simulink model "Closed_Loop_Simulation"  (R2022b)
settings: Solver=VariableStepAuto  StartTime=0.0  StopTime=100  RelTol=1e-3
values from neighbouring files (symbols this model uses):
  den = conv([2 1 0],[10 1])    [LAB03.m]    (also in StaticVelocityErrorConstant.m = [1 0])
  num = [2.5 5]    [LAB03.m]    (also in StaticVelocityErrorConstant.m = 5)
settings Model: Creator=Abdallah Awdallah  LastModifiedBy=Abdallah Awdallah

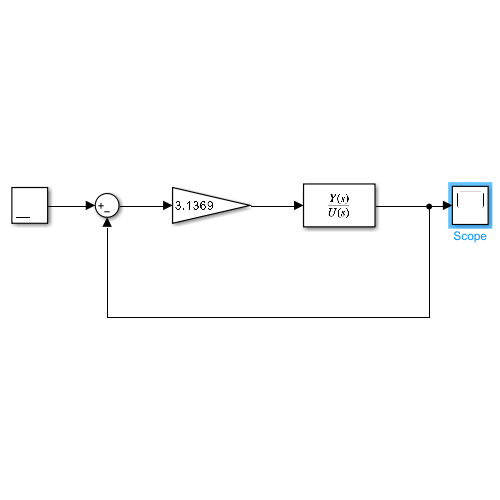
[thumbnail: Simulink's stored preview of the top-level diagram]
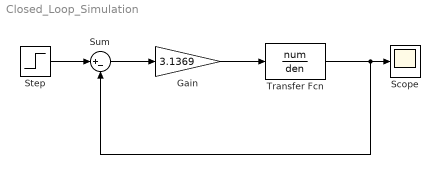
== system Closed_Loop_Simulation ==
  Gain : Gain  Gain=3.1369
  Scope : Scope
  Step : Step  Time=0  SampleTime=0
  Sum : Sum  Inputs=|+-
  Transfer Fcn : TransferFcn  Numerator=num  Denominator=den
  wires:
  Sum/1 -> Gain/1
  Gain/1 -> Transfer Fcn/1
  Transfer Fcn/1 -> Sum/2, Scope/1
  Step/1 -> Sum/1
